simulink model "gm_BilateralFilterIP"  (R2021a)
settings: Solver=FixedStepDiscrete  StartTime=0.0  StopTime=Ts_480p*5  RelTol=1e-3
InitFcn:
  | Ts = 1e-3;
  | Ts_240p = 402*324*Ts;
  | Ts_480p = 525*800*Ts;
undefined symbols (not defined in the file or in its folder): gray, Rec, SDTV
libraries: hdlsllib x8, visionhdlio x2, visionhdlfilter x1, visionhdlconversions x1, dspvision x1
settings Model: ModifiedByFormat=The MathWorks Inc.  Creator=The MathWorks, Inc.  LastModifiedBy=The MathWorks Inc.
settings SolverCC: AlgebraicLoopSolver=TrustRegion
settings DataIOCC: LimitDataPoints=on  SaveFormat=Array  SaveOutput=off  SaveTime=off  ReturnWorkspaceOutputs=off
settings OptimizationCC: BlockReduction=off  ConditionallyExecuteInputs=off  DefaultParameterBehavior=Inlined  LifeSpan=inf
settings DebuggingCC: AlgebraicLoopMsg=error  SolverPrmCheckMsg=warning  InheritedTsInSrcMsg=none  SingleTaskRateTransMsg=error  ParameterPrecisionLossMsg=none  AllowSymbolicDim=off  SFUnexpectedBacktrackingDiag=warning  SFNoUnconditionalDefaultTransitionDiag=warning  SFExecutionAtInitializationDiag=none  SFMachineParentedDataDiag=warning  IntegerSaturationMsg=none  ArithmeticOperatorsInVariantConditions=warning
settings HardwareCC: ProdBitPerPointer=32  ProdBitPerSizeT=32  ProdBitPerPtrDiffT=32  ProdLargestAtomicFloat=None  ProdIntDivRoundTo=Undefined  ProdEndianess=Unspecified  ProdWordSize=32  ProdHWDeviceType=ASIC/FPGA->ASIC/FPGA  ProdEqTarget=off
settings ModelReferenceCC: PropagateSignalLabelsOutOfModel=off
settings SFSimCC: SimUseLocalCustomCode=off  CustomCodeUndefinedFunction=UseInterfaceOnly
settings RTWCC: RTWUseLocalCustomCode=off
settings CodeAppCC: StateflowObjectComments=on
settings GRTTargetCC: TargetLangStandard=C89/C90 (ANSI)
settings ConfigComp: CovMetricSettings=dw  CovSaveCumulativeToWorkspaceVar=on  CovSaveSingleToWorkspaceVar=on  CovExternalEMLEnable=off  CovSFcnEnable=off

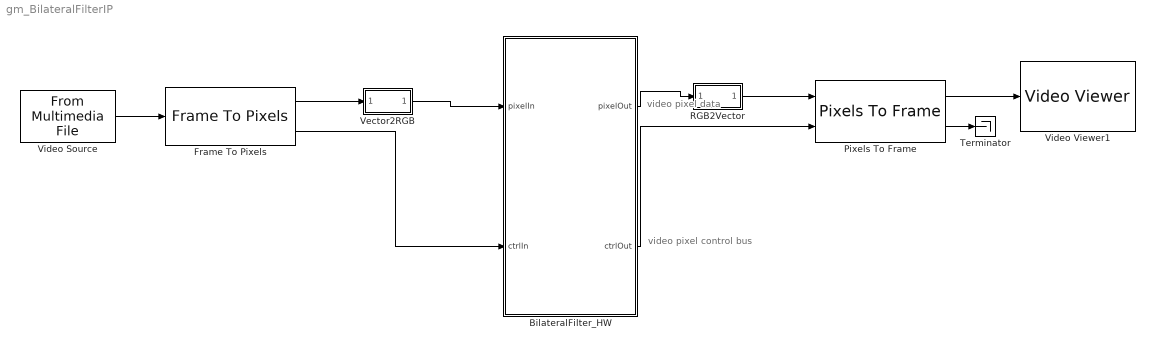
== system gm_BilateralFilterIP ==
  note: video pixel control bus
  note: video pixel data
  BilateralFilter_HW : Subsystem  TreatAsAtomicUnit=on
  Frame To Pixels : visionhdlio/Frame To Pixels  NumComponents=3  NumPixels=1  VideoFormat=480p  ActivePixelsPerLine=32  ActiveVideoLines=18  TotalPixelsPerLine=42  TotalVideoLines=28  StartingActiveLine=6  FrontPorch=5  SampleTime=0
      settings: SourceProductBaseCode=VT
  Pixels To Frame : visionhdlio/Pixels To Frame  NumComponents=3  NumPixels=1  VideoFormat=480p  ActivePixelsPerLine=32  ActiveVideoLines=18  TotalPixelsPerLine=42  TotalVideoLines=28
      settings: SourceProductBaseCode=VT
  RGB2Vector : Subsystem
  Terminator : Terminator
  Vector2RGB : Subsystem
  Video Source : dspvision/From Multimedia File  inputFilename=D:\Work\Custom_IP_Cores\Matlab\testImages\engine_480p.bmp  readRange=[1 Inf]  loop=on  numPlays=inf  outputStreams=Video only  videoDataType=uint8  audioDataType=int16  inheritSampleTime=off  userDefinedSampleTime=Ts_480p  noAudioOutput=off  isIntensityVideo=off  fourcc=RGB  colorVideoFormat=One multidimensional signal  outputEOF=off  dataOrg=Column-major  audioFrameSize=1024  computeAudioFrameSize=off  outSamplingMode=Sample based
  Video Viewer1 : VideoViewer  colormapValue=gray(256)  FigPos=[735 696 677 508]
  wires:
  BilateralFilter_HW/2(ctrlOut) -> Pixels To Frame/2
  Frame To Pixels/2 -> BilateralFilter_HW/2(ctrlIn)
  RGB2Vector/1(RGBVector) -> Pixels To Frame/1
  Frame To Pixels/1 -> Vector2RGB/1(RGBVector)
  Video Source/1 -> Frame To Pixels/1
  BilateralFilter_HW/1(pixelOut) -> RGB2Vector/1(RGB)
  Vector2RGB/1(RGB) -> BilateralFilter_HW/1(pixelIn)
  Pixels To Frame/1 -> Video Viewer1/1
  Pixels To Frame/2 -> Terminator/1

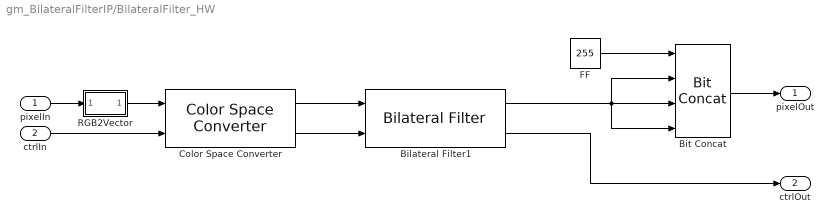
== system gm_BilateralFilterIP/BilateralFilter_HW ==
  pixelIn : Inport
  ctrlIn : Inport  Port=2
  Bilateral Filter1 : visionhdlfilter/Bilateral Filter  NeighborhoodSize=9x9  SpatialStdDev=3  IntensityStdDev=0.75  PaddingMethod=Replicate  PaddingValue=0  LineBufferSize=1024  SimulateUsing=Code generation  CoefficientsDataTypeStr=fixdt(0,22,22)  roundingMode=Nearest  overflowMode=on  OutputDataTypeStr=fixdt(0,8,0)  OutputMin=[]  OutputMax=[]
      settings: SourceProductBaseCode=VT
  Bit Concat : hdlsllib/Logic and Bit Operations/Bit Concat  numInputs=4
  Color Space Converter : visionhdlconversions/Color Space Converter  Conversion=RGB to intensity  ConversionStandard=Rec. 601 (SDTV)  ScanningStandard=1250/50/2:1  SimulateUsing=Code generation
      settings: SourceProductBaseCode=VT
  FF : Constant  Value=255  OutDataTypeStr=uint8  SampleTime=Ts
  RGB2Vector : Subsystem
  pixelOut : Outport  VectorParamsAs1DForOutWhenUnconnected=off
  ctrlOut : Outport  Port=2  VectorParamsAs1DForOutWhenUnconnected=off
  wires:
  Bilateral Filter1/2 -> ctrlOut/1
  Bilateral Filter1/1 -> Bit Concat/2, Bit Concat/3, Bit Concat/4
  Color Space Converter/2 -> Bilateral Filter1/2
  Color Space Converter/1 -> Bilateral Filter1/1
  Bit Concat/1 -> pixelOut/1
  FF/1 -> Bit Concat/1
  RGB2Vector/1(RGBVector) -> Color Space Converter/1
  pixelIn/1 -> RGB2Vector/1(RGB)
  ctrlIn/1 -> Color Space Converter/2

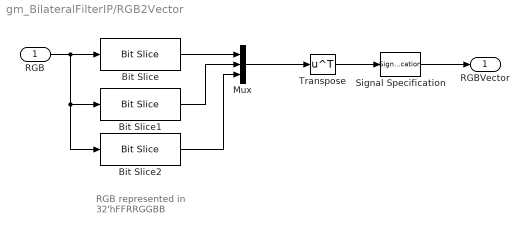
== system gm_BilateralFilterIP/RGB2Vector ==
  note: RGB represented in
      | 32'hFFRRGGBB
  RGB : Inport
  Bit Slice : hdlsllib/Logic and Bit Operations/Bit Slice  lidx=23  ridx=16
      settings: SourceProductBaseCode=SL
  Bit Slice1 : hdlsllib/Logic and Bit Operations/Bit Slice  lidx=15  ridx=8
      settings: SourceProductBaseCode=SL
  Bit Slice2 : hdlsllib/Logic and Bit Operations/Bit Slice  lidx=7  ridx=0
      settings: SourceProductBaseCode=SL
  Mux : Mux  Inputs=3
  Signal Specification : SignalSpecification
  Transpose : Math  Operator=transpose  SignedPower=on  SaturateOnIntegerOverflow=on
  RGBVector : Outport  VectorParamsAs1DForOutWhenUnconnected=off
  wires:
  Signal Specification/1 -> RGBVector/1
  Transpose/1 -> Signal Specification/1
  RGB/1 -> Bit Slice/1, Bit Slice1/1, Bit Slice2/1
  Bit Slice1/1 -> Mux/2
  Bit Slice2/1 -> Mux/3
  Bit Slice/1 -> Mux/1
  Mux/1 -> Transpose/1

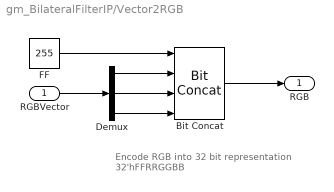
== system gm_BilateralFilterIP/Vector2RGB ==
  note: Encode RGB into 32 bit representation
      | 32'hFFRRGGBB
  RGBVector : Inport
  Bit Concat : hdlsllib/Logic and Bit Operations/Bit Concat  numInputs=4
  Demux : Demux  Outputs=3
  FF : Constant  Value=255  OutDataTypeStr=uint8  SampleTime=Ts
  RGB : Outport  VectorParamsAs1DForOutWhenUnconnected=off
  wires:
  Demux/3 -> Bit Concat/4
  Demux/2 -> Bit Concat/3
  Demux/1 -> Bit Concat/2
  FF/1 -> Bit Concat/1
  RGBVector/1 -> Demux/1
  Bit Concat/1 -> RGB/1

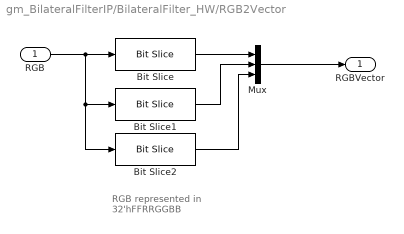
== system gm_BilateralFilterIP/BilateralFilter_HW/RGB2Vector ==
  note: RGB represented in
      | 32'hFFRRGGBB
  RGB : Inport
  Bit Slice : hdlsllib/Logic and Bit Operations/Bit Slice  lidx=23  ridx=16
      settings: SourceProductBaseCode=SL
  Bit Slice1 : hdlsllib/Logic and Bit Operations/Bit Slice  lidx=15  ridx=8
      settings: SourceProductBaseCode=SL
  Bit Slice2 : hdlsllib/Logic and Bit Operations/Bit Slice  lidx=7  ridx=0
      settings: SourceProductBaseCode=SL
  Mux : Mux  Inputs=3
  RGBVector : Outport  VectorParamsAs1DForOutWhenUnconnected=off
  wires:
  Mux/1 -> RGBVector/1
  RGB/1 -> Bit Slice/1, Bit Slice1/1, Bit Slice2/1
  Bit Slice1/1 -> Mux/2
  Bit Slice2/1 -> Mux/3
  Bit Slice/1 -> Mux/1
